simulink model "BST"  (R2023b)
settings: Solver=VariableStepAuto  StartTime=0.0  StopTime=10.0  RelTol=1e-3
libraries: simulink x31
settings Model: Creator=jsonm  LastModifiedBy=jsonm

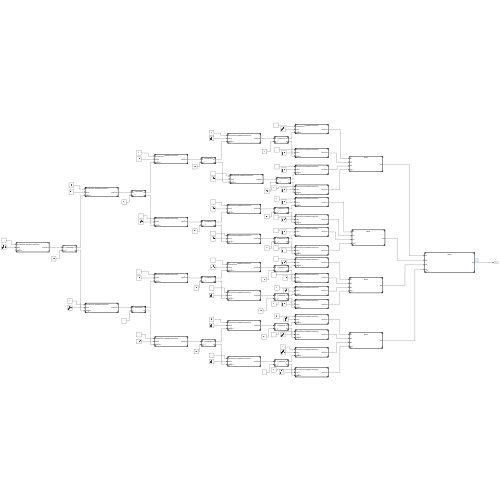
[thumbnail: Simulink's stored preview of the top-level diagram]
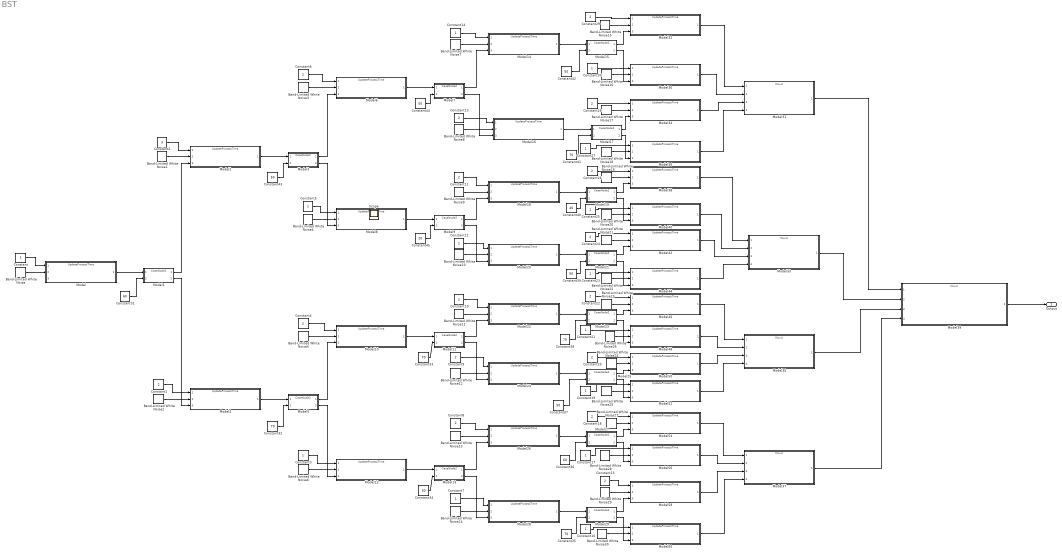
== system BST ==
  Band-Limited White Noise{,1..30} (31 alike) : simulink/Sources/Band-Limited White Noise  Cov=[0.1]  Ts=0.1  seed=[23341]
  Constant{,3,5,7,12,14,16..17,19,21,23,25,27,30} (14 alike) : Constant
  Constant{1,4,6,8..11,13,15,18,20,22,24,26,28..29} (16 alike) : Constant  Value=2
  Constant2 : Constant  Value=3
  Constant31 : Constant  Value=60
  Constant{32..33,35,38,41} (5 alike) : Constant  Value=70
  Constant34 : Constant  Value=30
  Constant36 : Constant  Value=60
  Constant{37,39,42..44} (5 alike) : Constant  Value=50
  Constant40 : Constant  Value=40
  Constant45 : Constant  Value=20
  Model{,2,4,6,8,10,12,14,16,18,20,22,24,26,28,30,32,34,36,38,40,42,44,46,48,50,52,54,56,58,60} (31 alike) : ModelReference  ModelNameDialog=UpdateProcessTime.slx  SimulationMode=Normal  ModelReferenceVersion=1.5
  Model{1,3,5,7,9,11,13,15,17,19,21,23,25,27,29} (15 alike) : ModelReference  ModelNameDialog=CaseNode2.slx  SimulationMode=Normal  ModelReferenceVersion=1.7
  Model{31,33,35,37,39} (5 alike) : ModelReference  ModelNameDialog=Mux4.slx  SimulationMode=Normal  ModelReferenceVersion=1.3
  Output : Outport
  Scope : Scope
  wires:
  Model/1 -> Model1/1
  Model2/1 -> Model3/1
  Model4/1 -> Model5/1
  Model6/1 -> Model7/1
  Model8/1 -> Model9/1
  Model10/1 -> Model11/1
  Model12/1 -> Model13/1
  Model14/1 -> Model15/1
  Model16/1 -> Model17/1
  Model18/1 -> Model19/1
  Model20/1 -> Model21/1
  Model22/1 -> Model23/1
  Model24/1 -> Model25/1
  Model26/1 -> Model27/1
  Model28/1 -> Model29/1
  Model30/1 -> Model31/2
  Model32/1 -> Model31/1
  Model34/1 -> Model31/3
  Model36/1 -> Model31/4
  Model38/1 -> Model33/1
  Model40/1 -> Model33/2
  Model42/1 -> Model33/3
  Model44/1 -> Model33/4
  Model46/1 -> Model35/1
  Model48/1 -> Model35/2
  Model50/1 -> Model35/3
  Model52/1 -> Model35/4
  Model54/1 -> Model37/1
  Model56/1 -> Model37/2
  Model58/1 -> Model37/3
  Model60/1 -> Model37/4
  Model3/1 -> Model6/3
  Model3/2 -> Model8/3
  Model7/1 -> Model14/3
  Model7/2 -> Model16/3
  Model9/1 -> Model18/3
  Model9/2 -> Model20/3
  Model15/1 -> Model32/3
  Model1/1 -> Model2/3
  Model1/2 -> Model4/3
  Model15/2 -> Model30/3
  Model17/1 -> Model34/3
  Model17/2 -> Model36/3
  Model19/1 -> Model38/3
  Model19/2 -> Model40/3
  Model21/1 -> Model42/3
  Model21/2 -> Model44/3
  Model23/1 -> Model46/3
  Model23/2 -> Model48/3
  Model25/1 -> Model50/3
  Model25/2 -> Model52/3
  Model27/1 -> Model54/3
  Model27/2 -> Model56/3
  Model29/1 -> Model58/3
  Model29/2 -> Model60/3
  Model13/1 -> Model26/3
  Model13/2 -> Model28/3
  Model11/1 -> Model22/3
  Model11/2 -> Model24/3
  Model5/1 -> Model10/3
  Model5/2 -> Model12/3
  Band-Limited White Noise/1 -> Model/2
  Band-Limited White Noise1/1 -> Model2/2
  Band-Limited White Noise2/1 -> Model4/2
  Band-Limited White Noise3/1 -> Model6/2
  Band-Limited White Noise4/1 -> Model8/2
  Band-Limited White Noise5/1 -> Model10/2
  Band-Limited White Noise6/1 -> Model12/2
  Band-Limited White Noise7/1 -> Model14/2
  Band-Limited White Noise8/1 -> Model16/2
  Band-Limited White Noise9/1 -> Model18/2
  Band-Limited White Noise10/1 -> Model20/2
  Band-Limited White Noise11/1 -> Model22/2
  Band-Limited White Noise12/1 -> Model24/2
  Band-Limited White Noise13/1 -> Model26/2
  Band-Limited White Noise14/1 -> Model28/2
  Band-Limited White Noise15/1 -> Model32/2
  Band-Limited White Noise16/1 -> Model30/2
  Band-Limited White Noise17/1 -> Model34/2
  Band-Limited White Noise18/1 -> Model36/2
  Band-Limited White Noise19/1 -> Model38/2
  Band-Limited White Noise20/1 -> Model40/2
  Band-Limited White Noise21/1 -> Model42/2
  Band-Limited White Noise22/1 -> Model44/2
  Band-Limited White Noise23/1 -> Model46/2
  Band-Limited White Noise24/1 -> Model50/2
  Band-Limited White Noise25/1 -> Model52/2
  Band-Limited White Noise26/1 -> Model48/2
  Band-Limited White Noise27/1 -> Model54/2
  Band-Limited White Noise28/1 -> Model56/2
  Band-Limited White Noise29/1 -> Model58/2
  Band-Limited White Noise30/1 -> Model60/2
  Constant/1 -> Model/1
  Constant1/1 -> Model4/1
  Constant2/1 -> Model2/1
  Constant3/1 -> Model12/1
  Constant4/1 -> Model10/1
  Constant5/1 -> Model8/1
  Constant6/1 -> Model6/1
  Constant7/1 -> Model28/1
  Constant8/1 -> Model26/1
  Constant9/1 -> Model24/1
  Constant10/1 -> Model22/1
  Constant11/1 -> Model18/1
  Constant12/1 -> Model20/1
  Constant13/1 -> Model16/1
  Constant14/1 -> Model14/1
  Constant15/1 -> Model58/1
  Constant16/1 -> Model60/1
  Constant17/1 -> Model56/1
  Constant18/1 -> Model54/1
  Constant19/1 -> Model52/1
  Constant20/1 -> Model50/1
  Constant21/1 -> Model48/1
  Constant22/1 -> Model46/1
  Constant23/1 -> Model44/1
  Constant24/1 -> Model42/1
  Constant25/1 -> Model40/1
  Constant26/1 -> Model38/1
  Constant27/1 -> Model36/1
  Constant28/1 -> Model34/1
  Constant29/1 -> Model32/1
  Constant30/1 -> Model30/1
  Constant31/1 -> Model1/2
  Constant32/1 -> Model5/2
  Constant33/1 -> Model11/2
  Constant34/1 -> Model13/2
  Constant35/1 -> Model29/2
  Constant36/1 -> Model27/2
  Constant37/1 -> Model25/2
  Constant38/1 -> Model23/2
  Constant39/1 -> Model21/2
  Constant40/1 -> Model19/2
  Constant41/1 -> Model17/2
  Constant42/1 -> Model15/2
  Constant43/1 -> Model3/2
  Constant44/1 -> Model7/2
  Constant45/1 -> Model9/2
  Model31/1 -> Model39/1
  Model33/1 -> Model39/2
  Model35/1 -> Model39/3
  Model37/1 -> Model39/4
  Model39/1 -> Output/1
